simulink library "slib_spectrum_analyser"  (R2020a)
settings: Solver=VariableStepAuto  StartTime=0.0  StopTime=10.0  RelTol=1e-3
libraries: hdlsllib x104, simulink x55, dsphdlxfrm x11, $bdroot x5
(part 1 of 3)
settings Model: Creator=david  LastModifiedBy=kevin

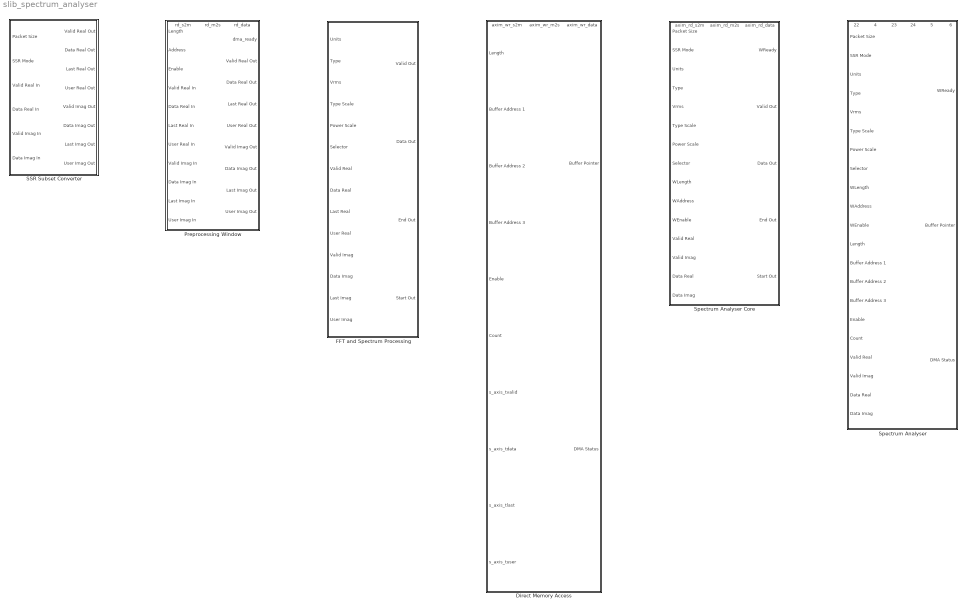
== system slib_spectrum_analyser ==
  Direct Memory Access : Subsystem  TreatAsAtomicUnit=on
      settings: PortSchema="{\"entries\":[{\"content\":{\"sides\":[{\"content\":{\"connectorIds\":[\"In1\",\"In2\",\"In3\",\"In4\",\"In5\",\"In6\",\"In7\",\"In8\",\"In9\",\"In10\"]},\"type\":\"ConnectorPlacement.EquallySpacedRectSide\",\"uuid\":\"feed7d54-868e-4051-a23d-06bc6ab36d5c\"},{\"content\":{\"connectorIds\":[\"Out1\",\"Out2\"],\"side\":\"RIGHT\"},\"type\":\"ConnectorPlacement.EquallySpacedRectSide\",\"uuid\":\"d3d03214-b2fe-4ae7-abfc-e707b28dda07\"},{\"content\":{\"connectorIds\":[\"In11\",\"Out3\",\"Out4\"],\"side\":\"TOP\"},\"type\":\"ConnectorPlacement.EquallySpacedRectSide\",\"uuid\":\"f475a445-5d90-4da5-970d-06e407d01a30\"}]},\"type\":\"ConnectorPlacement.EquallySpacedConnector\",\"uuid\":\"e5023fc6-91ea-4318-839d-5fb8d0ed3484\"}],\"packageUris\":[\"http://schema.mathworks.com/mf0/Connector/19700101\"],\"version\":\"1.0\"}"
  FFT and Spectrum Processing : Subsystem
  Preprocessing Window : Subsystem  TreatAsAtomicUnit=on
      settings: PortSchema="{\"entries\":[{\"content\":{\"sides\":[{\"content\":{\"connectorIds\":[\"In1\",\"In2\",\"In3\",\"In4\",\"In5\",\"In6\",\"In7\",\"In8\",\"In9\",\"In10\",\"In11\"]},\"type\":\"ConnectorPlacement.EquallySpacedRectSide\",\"uuid\":\"9bfde1a4-8e55-439d-ba95-b13ed8c2de82\"},{\"content\":{\"connectorIds\":[\"Out1\",\"Out2\",\"Out3\",\"Out4\",\"Out5\",\"Out6\",\"Out7\",\"Out8\",\"Out9\"],\"side\":\"RIGHT\"},\"type\":\"ConnectorPlacement.EquallySpacedRectSide\",\"uuid\":\"1fa858a7-8a79-448a-a9b9-a47438828a70\"},{\"content\":{\"connectorIds\":[\"In12\",\"Out10\",\"In13\"],\"side\":\"TOP\"},\"type\":\"ConnectorPlacement.EquallySpacedRectSide\",\"uuid\":\"fd991a14-ef2b-4cda-89a6-d580b9713fc0\"}]},\"type\":\"ConnectorPlacement.EquallySpacedConnector\",\"uuid\":\"ee399c2e-0a65-41c3-b55b-7131892126e8\"}],\"packageUris\":[\"http://schema.mathworks.com/mf0/Connector/19700101\"],\"version\":\"1.0\"}"
  SSR Subset Converter : Subsystem  TreatAsAtomicUnit=on
  Spectrum Analyser : Subsystem
      settings: PortSchema="{\"entries\":[{\"content\":{\"sides\":[{\"content\":{\"connectorIds\":[\"In1\",\"In2\",\"In3\",\"In4\",\"In5\",\"In6\",\"In7\",\"In8\",\"In9\",\"In10\",\"In11\",\"In12\",\"In13\",\"In14\",\"In15\",\"In16\",\"In17\",\"In18\",\"In19\",\"In20\",\"In21\"]},\"type\":\"ConnectorPlacement.EquallySpacedRectSide\",\"uuid\":\"d853649d-72ce-4bc9-937e-6765c6958e4b\"},{\"content\":{\"connectorIds\":[\"Out1\",\"Out2\",\"Out3\"],\"side\":\"RIGHT\"},\"type\":\"ConnectorPlacement.EquallySpacedRectSide\",\"uuid\":\"8ee09e61-17e3-46fa-8063-dedf2b48f93c\"},{\"content\":{\"connectorIds\":[\"In22\",\"Out4\",\"In23\",\"In24\",\"Out5\",\"Out6\"],\"side\":\"TOP\"},\"type\":\"ConnectorPlacement.EquallySpacedRectSide\",\"uuid\":\"c9845971-679e-4c10-9868-9337bdd39c3c\"}]},\"type\":\"ConnectorPlacement.EquallySpacedConnector\",\"uuid\":\"5955e85d-b605-4825-a1fe-b5d4f394d259\"}],\"packageUris\":[\"http://schema.mathworks.com/mf0/Connector/19700101\"],\"version\":\"1.0\"}"
  Spectrum Analyser Core : Subsystem
      settings: PortSchema="{\"entries\":[{\"content\":{\"sides\":[{\"content\":{\"connectorIds\":[\"In1\",\"In2\",\"In3\",\"In4\",\"In5\",\"In6\",\"In7\",\"In8\",\"In9\",\"In10\",\"In11\",\"In12\",\"In13\",\"In14\",\"In15\"]},\"type\":\"ConnectorPlacement.EquallySpacedRectSide\",\"uuid\":\"a616570c-2945-48d5-b176-114eb14b1374\"},{\"content\":{\"connectorIds\":[\"Out1\",\"Out2\",\"Out3\",\"Out4\",\"Out5\"],\"side\":\"RIGHT\"},\"type\":\"ConnectorPlacement.EquallySpacedRectSide\",\"uuid\":\"e19b5998-f051-43ca-87c3-ee1f351ddd7e\"},{\"content\":{\"connectorIds\":[\"In16\",\"Out6\",\"In17\"],\"side\":\"TOP\"},\"type\":\"ConnectorPlacement.EquallySpacedRectSide\",\"uuid\":\"3c8ee870-5dc0-4f24-aa51-29f9fa33db38\"}]},\"type\":\"ConnectorPlacement.EquallySpacedConnector\",\"uuid\":\"8f355573-d427-4bf9-9ede-a0a1ced230a6\"}],\"packageUris\":[\"http://schema.mathworks.com/mf0/Connector/19700101\"],\"version\":\"1.0\"}"

== system slib_spectrum_analyser/Direct Memory Access ==
  Length : Inport
  Buffer Address 1 : Inport  Port=2
  Buffer Address 2 : Inport  Port=3
  Buffer Address 3 : Inport  Port=4
  Enable : Inport  Port=5
  Count : Inport  Port=6
  s_axis_tvalid : Inport  Port=7
  s_axis_tdata : Inport  Port=8
  s_axis_tlast : Inport  Port=9
  s_axis_tuser : Inport  Port=10
  axim_wr_s2m : Inport  Port=11
  Direct Memory Access : Subsystem
      settings: PortSchema="{\"entries\":[{\"content\":{\"sides\":[{\"content\":{\"connectorIds\":[\"In1\",\"In2\",\"In3\",\"In4\",\"In5\",\"In6\",\"In7\",\"In8\",\"In9\",\"In10\"]},\"type\":\"ConnectorPlacement.EquallySpacedRectSide\",\"uuid\":\"00536163-74b2-48b0-a433-f45a47e82c13\"},{\"content\":{\"connectorIds\":[\"Out1\",\"Out2\",\"In11\",\"Out3\",\"Out4\",\"Out5\"],\"side\":\"RIGHT\"},\"type\":\"ConnectorPlacement.EquallySpacedRectSide\",\"uuid\":\"bb0450ed-1752-4cb2-9c7c-352c8b1a90c1\"},{\"content\":{\"connectorIds\":[],\"side\":\"TOP\"},\"type\":\"ConnectorPlacement.EquallySpacedRectSide\",\"uuid\":\"451bf01f-2efb-42e7-aace-9484eb9026e5\"}]},\"type\":\"ConnectorPlacement.EquallySpacedConnector\",\"uuid\":\"5c52148d-823b-46a6-a578-8e88341097d4\"}],\"packageUris\":[\"http://schema.mathworks.com/mf0/Connector/19700101\"],\"version\":\"1.0\"}"
  Terminator : Terminator
  Buffer Pointer : Outport
  DMA Status : Outport  Port=2
  axim_wr_m2s : Outport  Port=3
  axim_wr_data : Outport  Port=4
  wires:
  Direct Memory Access/5(debug_signals) -> Terminator/1
  Buffer Address 3/1 -> Direct Memory Access/5(Buffer Address 3)
  Buffer Address 2/1 -> Direct Memory Access/4(Buffer Address 2)
  Length/1 -> Direct Memory Access/1(Length)
  axim_wr_s2m/1 -> Direct Memory Access/11(wr_ready)
  Direct Memory Access/3(Buffer Pointer) -> Buffer Pointer/1
  Direct Memory Access/1(wr_data) -> axim_wr_data/1
  Enable/1 -> Direct Memory Access/6(Enable DMA)
  Buffer Address 1/1 -> Direct Memory Access/3(Buffer Address 1)
  Direct Memory Access/2(wr_m2s) -> axim_wr_m2s/1
  s_axis_tuser/1 -> Direct Memory Access/9(Start In)
  s_axis_tdata/1 -> Direct Memory Access/8(Data In)
  s_axis_tvalid/1 -> Direct Memory Access/7(Valid In)
  s_axis_tlast/1 -> Direct Memory Access/10(End In)
  Count/1 -> Direct Memory Access/2(Count)
  Direct Memory Access/4(DMA Status) -> DMA Status/1

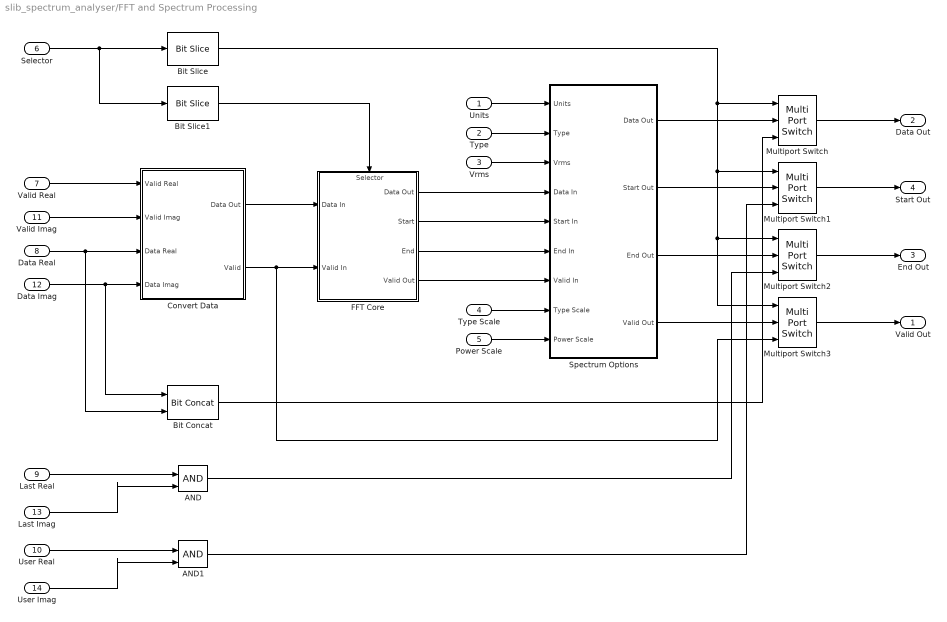
== system slib_spectrum_analyser/FFT and Spectrum Processing ==
  Units : Inport
  Type : Inport  Port=2
  Vrms : Inport  Port=3
  Type Scale : Inport  Port=4
  Power Scale : Inport  Port=5
  Selector : Inport  Port=6
  Valid Real : Inport  Port=7
  Data Real : Inport  Port=8
  Last Real : Inport  Port=9
  User Real : Inport  Port=10
  Valid Imag : Inport  Port=11
  Data Imag : Inport  Port=12
  Last Imag : Inport  Port=13
  User Imag : Inport  Port=14
  AND : Logic  IconShape=distinctive  AllPortsSameDT=off  OutDataTypeStr=boolean
  AND1 : Logic  IconShape=distinctive  AllPortsSameDT=off  OutDataTypeStr=boolean
  Bit Concat : hdlsllib/Logic and Bit Operations/Bit Concat  numInputs=2
  Bit Slice : hdlsllib/Logic and Bit Operations/Bit Slice  lidx=8  ridx=8
      settings: SourceProductBaseCode=SL
  Bit Slice1 : hdlsllib/Logic and Bit Operations/Bit Slice  lidx=7  ridx=0
      settings: SourceProductBaseCode=SL
  Convert Data : Subsystem
  FFT Core : Subsystem  VariantControl=FFT
      settings: PortSchema="{\"entries\":[{\"content\":{\"sides\":[{\"content\":{\"connectorIds\":[\"In1\",\"In2\"]},\"type\":\"ConnectorPlacement.EquallySpacedRectSide\",\"uuid\":\"5a82c6db-67e2-4b0c-874b-00e78ac3fdee\"},{\"content\":{\"connectorIds\":[\"Out1\",\"Out2\",\"Out3\",\"Out4\"],\"side\":\"RIGHT\"},\"type\":\"ConnectorPlacement.EquallySpacedRectSide\",\"uuid\":\"dd11d034-f57b-4257-86c3-a224676007d8\"},{\"content\":{\"connectorIds\":[\"In3\"],\"side\":\"TOP\"},\"type\":\"ConnectorPlacement.EquallySpacedRectSide\",\"uuid\":\"15a5b623-5fad-4b26-a0b8-0856d140e740\"}]},\"type\":\"ConnectorPlacement.EquallySpacedConnector\",\"uuid\":\"f1901d0a-924b-44ce-aa2b-38fba4da21f9\"}],\"packageUris\":[\"http://schema.mathworks.com/mf0/Connector/19700101\"],\"version\":\"1.0\"}"
  Multiport Switch{,1..3} (4 alike) : MultiPortSwitch  DataPortOrder=Zero-based contiguous  Inputs=2  zeroidx=on
  Spectrum Options : Subsystem  VariantControl=Options
  Valid Out : Outport
  Data Out : Outport  Port=2
  End Out : Outport  Port=3
  Start Out : Outport  Port=4
  wires:
  Bit Slice1/1 -> FFT Core/3(Selector)
  Bit Concat/1 -> Multiport Switch/3
  Vrms/1 -> Spectrum Options/3(Vrms)
  User Real/1 -> AND1/1
  Spectrum Options/2(Start Out) -> Multiport Switch1/2
  FFT Core/2(Start) -> Spectrum Options/5(Start In)
  AND/1 -> Multiport Switch2/3
  Spectrum Options/4(Valid Out) -> Multiport Switch3/2
  Last Imag/1 -> AND/2
  Multiport Switch3/1 -> Valid Out/1
  AND1/1 -> Multiport Switch1/3
  Multiport Switch/1 -> Data Out/1
  FFT Core/1(Data Out) -> Spectrum Options/4(Data In)
  Spectrum Options/3(End Out) -> Multiport Switch2/2
  Data Imag/1 -> Convert Data/4(Data Imag), Bit Concat/1
  Valid Real/1 -> Convert Data/1(Valid Real)
  Selector/1 -> Bit Slice/1, Bit Slice1/1
  Multiport Switch2/1 -> End Out/1
  Last Real/1 -> AND/1
  Multiport Switch1/1 -> Start Out/1
  Spectrum Options/1(Data Out) -> Multiport Switch/2
  Type Scale/1 -> Spectrum Options/8(Type Scale)
  Data Real/1 -> Convert Data/3(Data Real), Bit Concat/2
  FFT Core/4(Valid Out) -> Spectrum Options/7(Valid In)
  Power Scale/1 -> Spectrum Options/9(Power Scale)
  Convert Data/1(Data Out) -> FFT Core/1(Data In)
  Type/1 -> Spectrum Options/2(Type)
  User Imag/1 -> AND1/2
  Bit Slice/1 -> Multiport Switch/1, Multiport Switch1/1, Multiport Switch2/1, Multiport Switch3/1
  Units/1 -> Spectrum Options/1(Units)
  Valid Imag/1 -> Convert Data/2(Valid Imag)
  Convert Data/2(Valid) -> FFT Core/2(Valid In), Multiport Switch3/3
  FFT Core/3(End) -> Spectrum Options/6(End In)

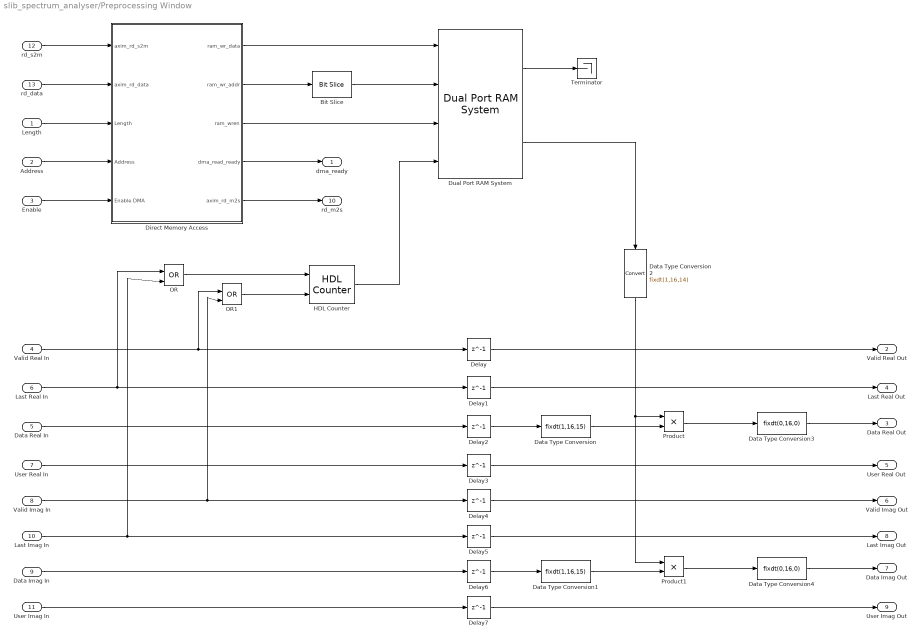
== system slib_spectrum_analyser/Preprocessing Window ==
  Length : Inport
  Address : Inport  Port=2
  Enable : Inport  Port=3
  Valid Real In : Inport  Port=4
  Data Real In : Inport  Port=5
  Last Real In : Inport  Port=6
  User Real In : Inport  Port=7
  Valid Imag In : Inport  Port=8
  Data Imag In : Inport  Port=9
  Last Imag In : Inport  Port=10
  User Imag In : Inport  Port=11
  rd_s2m : Inport  Port=12
  rd_data : Inport  Port=13
  Bit Slice : hdlsllib/Logic and Bit Operations/Bit Slice  lidx=12  ridx=0
      settings: SourceProductBaseCode=SL
  Data Type Conversion : DataTypeConversion  OutDataTypeStr=fixdt(1,16,15)  ConvertRealWorld=Stored Integer (SI)
  Data Type Conversion1 : DataTypeConversion  OutDataTypeStr=fixdt(1,16,15)  ConvertRealWorld=Stored Integer (SI)
  Data Type Conversion2 : DataTypeConversion  OutDataTypeStr=fixdt(1,16,14)  ConvertRealWorld=Stored Integer (SI)
  Data Type Conversion3 : DataTypeConversion  OutDataTypeStr=fixdt(0,16,0)  ConvertRealWorld=Stored Integer (SI)
  Data Type Conversion4 : DataTypeConversion  OutDataTypeStr=fixdt(0,16,0)  ConvertRealWorld=Stored Integer (SI)
  Delay{,1..7} (8 alike) : Delay  DelayLength=1
  Direct Memory Access : Subsystem
  Dual Port RAM System : hdlsllib/HDL RAMs/Dual Port RAM System  RAMType=Dual port  WriteOutputValue=New data  RAMInitialValue=ones(1, 2^13)*2^14  SimulateUsing=Code generation
      settings: SourceProductBaseCode=SL
  HDL Counter : hdlsllib/Sources/HDL Counter  CountType=Count limited  CountInit=0  CountStep=1  CountMax=8191  CountFromType=Initial value  CountFrom=0  CountResetPort=on  CountLoadPort=off  CountEnbPort=on  CountDirPort=off  CountDataType=Unsigned  CountWordLen=13  CountFracLen=0  CountSampTime=1
  OR : Logic  Operator=OR  IconShape=distinctive  AllPortsSameDT=off  OutDataTypeStr=boolean
  OR1 : Logic  Operator=OR  IconShape=distinctive  AllPortsSameDT=off  OutDataTypeStr=boolean
  Product : Product  OutDataTypeStr=fixdt(1,16,15)  RndMeth=Round  SaturateOnIntegerOverflow=on
  Product1 : Product  OutDataTypeStr=fixdt(1,16,15)  RndMeth=Round  SaturateOnIntegerOverflow=on
  Terminator : Terminator
  dma_ready : Outport
  Valid Real Out : Outport  Port=2
  Data Real Out : Outport  Port=3
  Last Real Out : Outport  Port=4
  User Real Out : Outport  Port=5
  Valid Imag Out : Outport  Port=6
  Data Imag Out : Outport  Port=7
  Last Imag Out : Outport  Port=8
  User Imag Out : Outport  Port=9
  rd_m2s : Outport  Port=10
  wires:
  Address/1 -> Direct Memory Access/4(Address)
  Enable/1 -> Direct Memory Access/5(Enable DMA)
  Length/1 -> Direct Memory Access/3(Length)
  Direct Memory Access/1(ram_wr_data) -> Dual Port RAM System/1
  Direct Memory Access/2(ram_wr_addr) -> Bit Slice/1
  Direct Memory Access/3(ram_wren) -> Dual Port RAM System/3
  Direct Memory Access/4(dma_read_ready) -> dma_ready/1
  HDL Counter/1 -> Dual Port RAM System/4
  Valid Real In/1 -> OR1/1, Delay/1
  Last Real In/1 -> OR/1, Delay1/1
  Dual Port RAM System/1 -> Terminator/1
  Direct Memory Access/5(axim_rd_m2s) -> rd_m2s/1
  Dual Port RAM System/2 -> Data Type Conversion2/1
  Data Real In/1 -> Delay2/1
  Product/1 -> Data Type Conversion3/1
  User Real In/1 -> Delay3/1
  OR/1 -> HDL Counter/1
  OR1/1 -> HDL Counter/2
  Last Imag In/1 -> OR/2, Delay5/1
  Valid Imag In/1 -> OR1/2, Delay4/1
  Data Imag In/1 -> Delay6/1
  Product1/1 -> Data Type Conversion4/1
  User Imag In/1 -> Delay7/1
  rd_s2m/1 -> Direct Memory Access/1(axim_rd_s2m)
  rd_data/1 -> Direct Memory Access/2(axim_rd_data)
  Data Type Conversion/1 -> Product/2
  Data Type Conversion1/1 -> Product1/2
  Data Type Conversion2/1 -> Product1/1, Product/1
  Data Type Conversion3/1 -> Data Real Out/1
  Data Type Conversion4/1 -> Data Imag Out/1
  Delay/1 -> Valid Real Out/1
  Delay1/1 -> Last Real Out/1
  Delay2/1 -> Data Type Conversion/1
  Delay3/1 -> User Real Out/1
  Delay4/1 -> Valid Imag Out/1
  Delay5/1 -> Last Imag Out/1
  Delay6/1 -> Data Type Conversion1/1
  Delay7/1 -> User Imag Out/1
  Bit Slice/1 -> Dual Port RAM System/2

== system slib_spectrum_analyser/SSR Subset Converter ==
  Packet Size : Inport
  SSR Mode : Inport  Port=2
  Valid Real In : Inport  Port=3
  Data Real In : Inport  Port=4
  Valid Imag In : Inport  Port=5
  Data Imag In : Inport  Port=6
  Bit Slice : hdlsllib/Logic and Bit Operations/Bit Slice  lidx=3  ridx=0
      settings: SourceProductBaseCode=SL
  SSR Deserializer Imag : Subsystem
  SSR Deserializer Real : Subsystem
  SSR Packet Generator Imag : Subsystem
      settings: PortSchema="{\"entries\":[{\"content\":{\"sides\":[{\"content\":{\"connectorIds\":[\"In1\",\"In2\",\"In3\"]},\"type\":\"ConnectorPlacement.EquallySpacedRectSide\",\"uuid\":\"a59bbe9b-b017-421a-b59e-ccf8f0be8c6c\"},{\"content\":{\"connectorIds\":[\"Out1\",\"Out2\",\"Out3\",\"Out4\"],\"side\":\"RIGHT\"},\"type\":\"ConnectorPlacement.EquallySpacedRectSide\",\"uuid\":\"db28a192-666b-40ba-a3e6-dc552d532719\"},{\"content\":{\"connectorIds\":[\"In4\"],\"side\":\"TOP\"},\"type\":\"ConnectorPlacement.EquallySpacedRectSide\",\"uuid\":\"3e188adb-8196-4c2d-ad94-9c10f40ece47\"}]},\"type\":\"ConnectorPlacement.EquallySpacedConnector\",\"uuid\":\"a5800336-434d-4feb-8784-3c17a141dc8c\"}],\"packageUris\":[\"http://schema.mathworks.com/mf0/Connector/19700101\"],\"version\":\"1.0\"}"
  SSR Packet Generator Real : Subsystem
      settings: PortSchema="{\"entries\":[{\"content\":{\"sides\":[{\"content\":{\"connectorIds\":[\"In1\",\"In2\",\"In3\"]},\"type\":\"ConnectorPlacement.EquallySpacedRectSide\",\"uuid\":\"a59bbe9b-b017-421a-b59e-ccf8f0be8c6c\"},{\"content\":{\"connectorIds\":[\"Out1\",\"Out2\",\"Out3\",\"Out4\"],\"side\":\"RIGHT\"},\"type\":\"ConnectorPlacement.EquallySpacedRectSide\",\"uuid\":\"db28a192-666b-40ba-a3e6-dc552d532719\"},{\"content\":{\"connectorIds\":[\"In4\"],\"side\":\"TOP\"},\"type\":\"ConnectorPlacement.EquallySpacedRectSide\",\"uuid\":\"3e188adb-8196-4c2d-ad94-9c10f40ece47\"}]},\"type\":\"ConnectorPlacement.EquallySpacedConnector\",\"uuid\":\"a5800336-434d-4feb-8784-3c17a141dc8c\"}],\"packageUris\":[\"http://schema.mathworks.com/mf0/Connector/19700101\"],\"version\":\"1.0\"}"
  SSR Serializer Imag : Subsystem
  SSR Serializer Real : Subsystem
  Valid Real Out : Outport
  Data Real Out : Outport  Port=2
  Last Real Out : Outport  Port=3
  User Real Out : Outport  Port=4
  Valid Imag Out : Outport  Port=5
  Data Imag Out : Outport  Port=6
  Last Imag Out : Outport  Port=7
  User Imag Out : Outport  Port=8
  wires:
  SSR Serializer Real/2(Data Out) -> SSR Packet Generator Real/3(Data In)
  SSR Packet Generator Real/4(EoF Out) -> SSR Deserializer Real/4(EoF In)
  Data Real In/1 -> SSR Serializer Real/3(Data In)
  SSR Serializer Real/1(Valid Out) -> SSR Packet Generator Real/2(Valid In)
  SSR Deserializer Real/3(SoF Out) -> User Real Out/1
  Bit Slice/1 -> SSR Serializer Real/1(SSR Control), SSR Serializer Imag/1(SSR Control), SSR Packet Generator Real/1(Frame Drop), SSR Packet Generator Imag/1(Frame Drop)
  SSR Packet Generator Real/1(Valid Out) -> SSR Deserializer Real/1(Valid In)
  Valid Real In/1 -> SSR Serializer Real/2(Valid In)
  SSR Packet Generator Real/3(SoF Out) -> SSR Deserializer Real/3(SoF In)
  SSR Packet Generator Real/2(Data Out) -> SSR Deserializer Real/2(Data In)
  SSR Deserializer Real/2(Data Out) -> Data Real Out/1
  SSR Mode/1 -> Bit Slice/1
  SSR Deserializer Real/1(Valid Out) -> Valid Real Out/1
  SSR Deserializer Real/4(EoL Out) -> Last Real Out/1
  Packet Size/1 -> SSR Packet Generator Real/4(Packet Size), SSR Packet Generator Imag/4(Packet Size)
  Valid Imag In/1 -> SSR Serializer Imag/2(Valid In)
  Data Imag In/1 -> SSR Serializer Imag/3(Data In)
  SSR Serializer Imag/1(Valid Out) -> SSR Packet Generator Imag/2(Valid In)
  SSR Serializer Imag/2(Data Out) -> SSR Packet Generator Imag/3(Data In)
  SSR Deserializer Imag/4(EoL Out) -> Last Imag Out/1
  SSR Deserializer Imag/1(Valid Out) -> Valid Imag Out/1
  SSR Deserializer Imag/2(Data Out) -> Data Imag Out/1
  SSR Deserializer Imag/3(SoF Out) -> User Imag Out/1
  SSR Packet Generator Imag/1(Valid Out) -> SSR Deserializer Imag/1(Valid In)
  SSR Packet Generator Imag/2(Data Out) -> SSR Deserializer Imag/2(Data In)
  SSR Packet Generator Imag/3(SoF Out) -> SSR Deserializer Imag/3(SoF In)
  SSR Packet Generator Imag/4(EoF Out) -> SSR Deserializer Imag/4(EoF In)

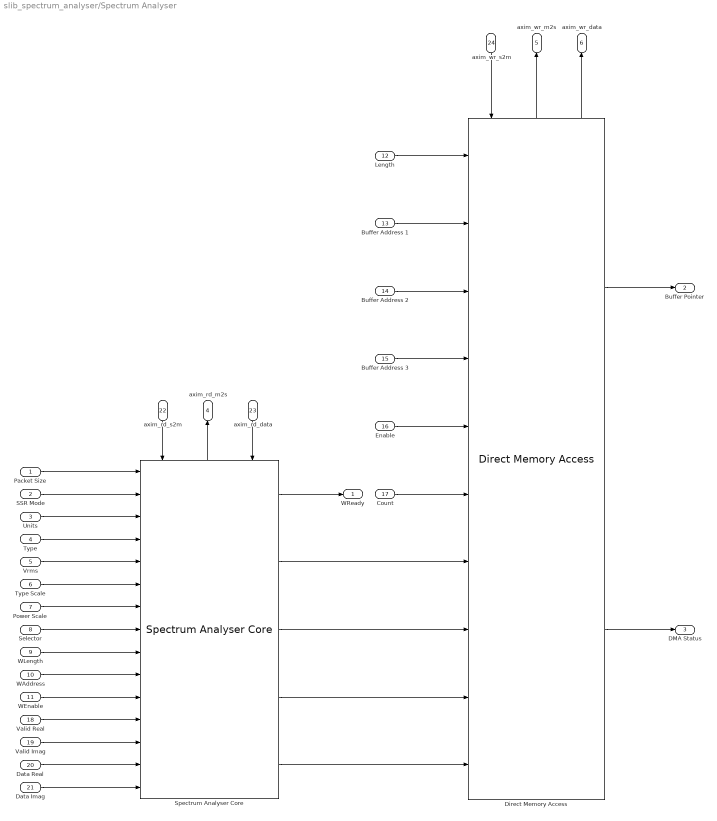
== system slib_spectrum_analyser/Spectrum Analyser ==
  Packet Size : Inport
  SSR Mode : Inport  Port=2
  Units : Inport  Port=3
  Type : Inport  Port=4
  Vrms : Inport  Port=5
  Type Scale : Inport  Port=6
  Power Scale : Inport  Port=7
  Selector : Inport  Port=8
  WLength : Inport  Port=9
  WAddress : Inport  Port=10
  WEnable : Inport  Port=11
  Length : Inport  Port=12
  Buffer Address 1 : Inport  Port=13
  Buffer Address 2 : Inport  Port=14
  Buffer Address 3 : Inport  Port=15
  Enable : Inport  Port=16
  Count : Inport  Port=17
  Valid Real : Inport  Port=18
  Valid Imag : Inport  Port=19
  Data Real : Inport  Port=20
  Data Imag : Inport  Port=21
  axim_rd_s2m : Inport  Port=22
  axim_rd_data : Inport  Port=23
  axim_wr_s2m : Inport  Port=24
  Direct Memory Access : $bdroot/Direct Memory Access  SystemSampleTime=-1  Latency=0  AutoFrameSizeCalculation=off
      settings: PortSchema="{\"entries\":[{\"content\":{\"sides\":[{\"content\":{\"connectorIds\":[\"In1\",\"In2\",\"In3\",\"In4\",\"In5\",\"In6\",\"In7\",\"In8\",\"In9\",\"In10\"]},\"type\":\"ConnectorPlacement.EquallySpacedRectSide\",\"uuid\":\"feed7d54-868e-4051-a23d-06bc6ab36d5c\"},{\"content\":{\"connectorIds\":[\"Out1\",\"Out2\"],\"side\":\"RIGHT\"},\"type\":\"ConnectorPlacement.EquallySpacedRectSide\",\"uuid\":\"d3d03214-b2fe-4ae7-abfc-e707b28dda07\"},{\"content\":{\"connectorIds\":[\"In11\",\"Out3\",\"Out4\"],\"side\":\"TOP\"},\"type\":\"ConnectorPlacement.EquallySpacedRectSide\",\"uuid\":\"f475a445-5d90-4da5-970d-06e407d01a30\"}]},\"type\":\"ConnectorPlacement.EquallySpacedConnector\",\"uuid\":\"e5023fc6-91ea-4318-839d-5fb8d0ed3484\"}],\"packageUris\":[\"http://schema.mathworks.com/mf0/Connector/19700101\"],\"version\":\"1.0\"}"
  Spectrum Analyser Core : $bdroot/Spectrum Analyser Core  SystemSampleTime=-1  Latency=0  AutoFrameSizeCalculation=off
      settings: PortSchema="{\"entries\":[{\"content\":{\"sides\":[{\"content\":{\"connectorIds\":[\"In1\",\"In2\",\"In3\",\"In4\",\"In5\",\"In6\",\"In7\",\"In8\",\"In9\",\"In10\",\"In11\",\"In12\",\"In13\",\"In14\",\"In15\"]},\"type\":\"ConnectorPlacement.EquallySpacedRectSide\",\"uuid\":\"a616570c-2945-48d5-b176-114eb14b1374\"},{\"content\":{\"connectorIds\":[\"Out1\",\"Out2\",\"Out3\",\"Out4\",\"Out5\"],\"side\":\"RIGHT\"},\"type\":\"ConnectorPlacement.EquallySpacedRectSide\",\"uuid\":\"e19b5998-f051-43ca-87c3-ee1f351ddd7e\"},{\"content\":{\"connectorIds\":[\"In16\",\"Out6\",\"In17\"],\"side\":\"TOP\"},\"type\":\"ConnectorPlacement.EquallySpacedRectSide\",\"uuid\":\"3c8ee870-5dc0-4f24-aa51-29f9fa33db38\"}]},\"type\":\"ConnectorPlacement.EquallySpacedConnector\",\"uuid\":\"8f355573-d427-4bf9-9ede-a0a1ced230a6\"}],\"packageUris\":[\"http://schema.mathworks.com/mf0/Connector/19700101\"],\"version\":\"1.0\"}"
  WReady : Outport
  Buffer Pointer : Outport  Port=2
  DMA Status : Outport  Port=3
  axim_rd_m2s : Outport  Port=4
  axim_wr_m2s : Outport  Port=5
  axim_wr_data : Outport  Port=6
  wires:
  Direct Memory Access/3 -> axim_wr_m2s/1
  Spectrum Analyser Core/5 -> Direct Memory Access/10
  Spectrum Analyser Core/4 -> Direct Memory Access/9
  axim_rd_data/1 -> Spectrum Analyser Core/17
  Spectrum Analyser Core/3 -> Direct Memory Access/8
  Enable/1 -> Direct Memory Access/5
  axim_rd_s2m/1 -> Spectrum Analyser Core/16
  Spectrum Analyser Core/2 -> Direct Memory Access/7
  WEnable/1 -> Spectrum Analyser Core/11
  Data Imag/1 -> Spectrum Analyser Core/15
  Units/1 -> Spectrum Analyser Core/3
  WAddress/1 -> Spectrum Analyser Core/10
  Spectrum Analyser Core/1 -> WReady/1
  Power Scale/1 -> Spectrum Analyser Core/7
  Buffer Address 1/1 -> Direct Memory Access/2
  Type Scale/1 -> Spectrum Analyser Core/6
  Valid Real/1 -> Spectrum Analyser Core/12
  WLength/1 -> Spectrum Analyser Core/9
  Selector/1 -> Spectrum Analyser Core/8
  Type/1 -> Spectrum Analyser Core/4
  axim_wr_s2m/1 -> Direct Memory Access/11
  Direct Memory Access/4 -> axim_wr_data/1
  Packet Size/1 -> Spectrum Analyser Core/1
  Data Real/1 -> Spectrum Analyser Core/14
  Buffer Address 3/1 -> Direct Memory Access/4
  Direct Memory Access/2 -> DMA Status/1
  Direct Memory Access/1 -> Buffer Pointer/1
  Count/1 -> Direct Memory Access/6
  Spectrum Analyser Core/6 -> axim_rd_m2s/1
  Buffer Address 2/1 -> Direct Memory Access/3
  Length/1 -> Direct Memory Access/1
  SSR Mode/1 -> Spectrum Analyser Core/2
  Vrms/1 -> Spectrum Analyser Core/5
  Valid Imag/1 -> Spectrum Analyser Core/13

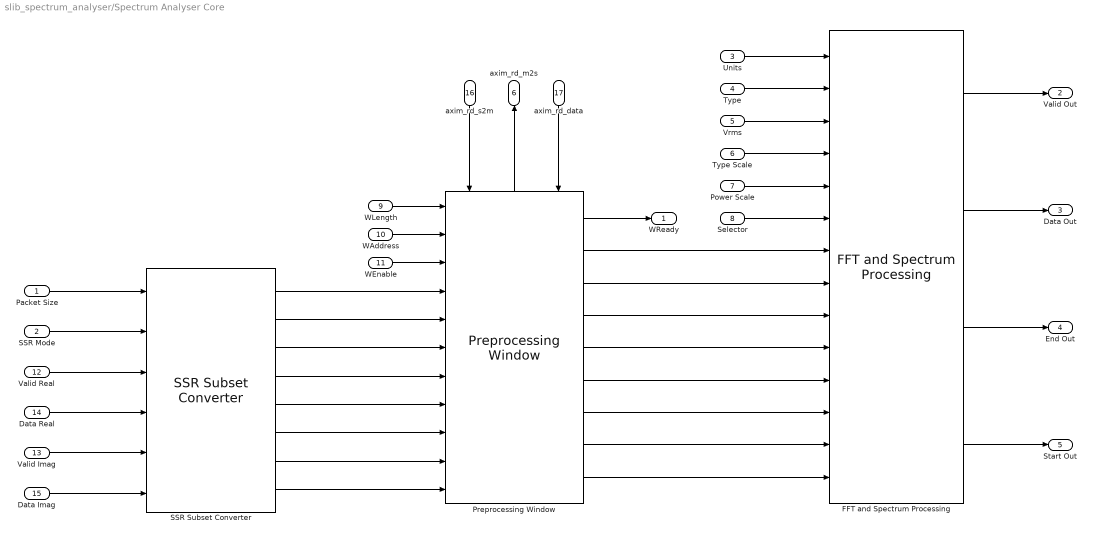
== system slib_spectrum_analyser/Spectrum Analyser Core ==
  Packet Size : Inport
  SSR Mode : Inport  Port=2
  Units : Inport  Port=3
  Type : Inport  Port=4
  Vrms : Inport  Port=5
  Type Scale : Inport  Port=6
  Power Scale : Inport  Port=7
  Selector : Inport  Port=8
  WLength : Inport  Port=9
  WAddress : Inport  Port=10
  WEnable : Inport  Port=11
  Valid Real : Inport  Port=12
  Valid Imag : Inport  Port=13
  Data Real : Inport  Port=14
  Data Imag : Inport  Port=15
  axim_rd_s2m : Inport  Port=16
  axim_rd_data : Inport  Port=17
  FFT and Spectrum Processing : $bdroot/FFT and Spectrum Processing  SystemSampleTime=-1  Latency=0  AutoFrameSizeCalculation=off
  Preprocessing Window : $bdroot/Preprocessing Window  SystemSampleTime=-1  Latency=0  AutoFrameSizeCalculation=off
      settings: PortSchema="{\"entries\":[{\"content\":{\"sides\":[{\"content\":{\"connectorIds\":[\"In1\",\"In2\",\"In3\",\"In4\",\"In5\",\"In6\",\"In7\",\"In8\",\"In9\",\"In10\",\"In11\"]},\"type\":\"ConnectorPlacement.EquallySpacedRectSide\",\"uuid\":\"9bfde1a4-8e55-439d-ba95-b13ed8c2de82\"},{\"content\":{\"connectorIds\":[\"Out1\",\"Out2\",\"Out3\",\"Out4\",\"Out5\",\"Out6\",\"Out7\",\"Out8\",\"Out9\"],\"side\":\"RIGHT\"},\"type\":\"ConnectorPlacement.EquallySpacedRectSide\",\"uuid\":\"1fa858a7-8a79-448a-a9b9-a47438828a70\"},{\"content\":{\"connectorIds\":[\"In12\",\"Out10\",\"In13\"],\"side\":\"TOP\"},\"type\":\"ConnectorPlacement.EquallySpacedRectSide\",\"uuid\":\"fd991a14-ef2b-4cda-89a6-d580b9713fc0\"}]},\"type\":\"ConnectorPlacement.EquallySpacedConnector\",\"uuid\":\"ee399c2e-0a65-41c3-b55b-7131892126e8\"}],\"packageUris\":[\"http://schema.mathworks.com/mf0/Connector/19700101\"],\"version\":\"1.0\"}"
  SSR Subset Converter : $bdroot/SSR Subset Converter  SystemSampleTime=-1  Latency=0  AutoFrameSizeCalculation=off
  WReady : Outport
  Valid Out : Outport  Port=2
  Data Out : Outport  Port=3
  End Out : Outport  Port=4
  Start Out : Outport  Port=5
  axim_rd_m2s : Outport  Port=6
  wires:
  Valid Imag/1 -> SSR Subset Converter/5
  Preprocessing Window/5 -> FFT and Spectrum Processing/10
  Preprocessing Window/1 -> WReady/1
  SSR Subset Converter/7 -> Preprocessing Window/10
  WEnable/1 -> Preprocessing Window/3
  Valid Real/1 -> SSR Subset Converter/3
  SSR Subset Converter/6 -> Preprocessing Window/9
  FFT and Spectrum Processing/2 -> Data Out/1
  axim_rd_data/1 -> Preprocessing Window/13
  Units/1 -> FFT and Spectrum Processing/1
  Preprocessing Window/8 -> FFT and Spectrum Processing/13
  FFT and Spectrum Processing/1 -> Valid Out/1
  Preprocessing Window/6 -> FFT and Spectrum Processing/11
  SSR Subset Converter/3 -> Preprocessing Window/6
  axim_rd_s2m/1 -> Preprocessing Window/12
  SSR Subset Converter/8 -> Preprocessing Window/11
  WLength/1 -> Preprocessing Window/1
  FFT and Spectrum Processing/3 -> End Out/1
  Data Real/1 -> SSR Subset Converter/4
  Preprocessing Window/7 -> FFT and Spectrum Processing/12
  SSR Mode/1 -> SSR Subset Converter/2
  Data Imag/1 -> SSR Subset Converter/6
  SSR Subset Converter/4 -> Preprocessing Window/7
  Power Scale/1 -> FFT and Spectrum Processing/5
  Preprocessing Window/4 -> FFT and Spectrum Processing/9
  SSR Subset Converter/5 -> Preprocessing Window/8
  Type/1 -> FFT and Spectrum Processing/2
  Vrms/1 -> FFT and Spectrum Processing/3
  Preprocessing Window/2 -> FFT and Spectrum Processing/7
  Selector/1 -> FFT and Spectrum Processing/6
  FFT and Spectrum Processing/4 -> Start Out/1
  Type Scale/1 -> FFT and Spectrum Processing/4
  WAddress/1 -> Preprocessing Window/2
  SSR Subset Converter/2 -> Preprocessing Window/5
  Preprocessing Window/9 -> FFT and Spectrum Processing/14
  Preprocessing Window/10 -> axim_rd_m2s/1
  SSR Subset Converter/1 -> Preprocessing Window/4
  Preprocessing Window/3 -> FFT and Spectrum Processing/8
  Packet Size/1 -> SSR Subset Converter/1

== system slib_spectrum_analyser/Direct Memory Access/Direct Memory Access ==
  Length : Inport
  Count : Inport  Port=2
  Buffer Address 1 : Inport  Port=3
  Buffer Address 2 : Inport  Port=4
  Buffer Address 3 : Inport  Port=5
  Enable DMA : Inport  Port=6
  Valid In : Inport  Port=7
  Data In : Inport  Port=8
  Start In : Inport  Port=9
  End In : Inport  Port=10
  wr_ready : Inport  Port=11
  DDR Communication : Subsystem
      settings: PortSchema="{\"entries\":[{\"content\":{\"sides\":[{\"content\":{\"connectorIds\":[\"In1\",\"In2\",\"In3\",\"In4\",\"In5\",\"In6\",\"In7\",\"In8\",\"In9\",\"In10\"]},\"type\":\"ConnectorPlacement.EquallySpacedRectSide\",\"uuid\":\"1b0605ed-f994-4b4f-952c-c7a4534a55db\"},{\"content\":{\"connectorIds\":[\"Out1\",\"Out2\",\"Out3\",\"Out4\",\"Out5\",\"In11\"],\"side\":\"RIGHT\"},\"type\":\"ConnectorPlacement.EquallySpacedRectSide\",\"uuid\":\"e00ce3f0-150b-4c4f-a18d-f280380b0728\"},{\"content\":{\"connectorIds\":[],\"side\":\"TOP\"},\"type\":\"ConnectorPlacement.EquallySpacedRectSide\",\"uuid\":\"b0ef8b1e-3f6b-405f-8824-c1fb25b076ef\"}]},\"type\":\"ConnectorPlacement.EquallySpacedConnector\",\"uuid\":\"53c75551-9c59-440c-835f-2065b8683bc1\"}],\"packageUris\":[\"http://schema.mathworks.com/mf0/Connector/19700101\"],\"version\":\"1.0\"}"
  wr_data : Outport
  wr_m2s : Outport  Port=2
  Buffer Pointer : Outport  Port=3
  DMA Status : Outport  Port=4
  debug_signals : Outport  Port=5
  wires:
  wr_ready/1 -> DDR Communication/11(wr_ready)
  DDR Communication/2(wr_data) -> wr_data/1
  DDR Communication/3(wr_m2s) -> wr_m2s/1
  Start In/1 -> DDR Communication/9(Start In)
  End In/1 -> DDR Communication/10(End In)
  Data In/1 -> DDR Communication/8(Data Out)
  DDR Communication/1(Buffer Pointer) -> Buffer Pointer/1
  Valid In/1 -> DDR Communication/7(Valid Out)
  Buffer Address 1/1 -> DDR Communication/3(Buffer Address 1)
  Buffer Address 2/1 -> DDR Communication/4(Buffer Address 2)
  Buffer Address 3/1 -> DDR Communication/5(Buffer Address 3)
  Enable DMA/1 -> DDR Communication/6(Enable)
  DDR Communication/4(DMA Status) -> DMA Status/1
  Length/1 -> DDR Communication/1(Length)
  DDR Communication/5(debug_signals) -> debug_signals/1
  Count/1 -> DDR Communication/2(Count)

== system slib_spectrum_analyser/FFT and Spectrum Processing/Convert Data ==
  Valid Real : Inport
  Valid Imag : Inport  Port=2
  Data Real : Inport  Port=3
  Data Imag : Inport  Port=4
  AND : Logic  IconShape=distinctive  AllPortsSameDT=off  OutDataTypeStr=boolean
  Data Type Conversion : DataTypeConversion  OutDataTypeStr=fixdt(1,16,15)  ConvertRealWorld=Stored Integer (SI)
  Data Type Conversion1 : DataTypeConversion  OutDataTypeStr=fixdt(1,16,15)  ConvertRealWorld=Stored Integer (SI)
  Real-Imag to Complex : RealImagToComplex
  Data Out : Outport
  Valid : Outport  Port=2
  wires:
  Valid Imag/1 -> AND/2
  Data Type Conversion1/1 -> Real-Imag to Complex/2
  Data Real/1 -> Data Type Conversion/1
  Data Type Conversion/1 -> Real-Imag to Complex/1
  Data Imag/1 -> Data Type Conversion1/1
  Valid Real/1 -> AND/1
  AND/1 -> Valid/1
  Real-Imag to Complex/1 -> Data Out/1

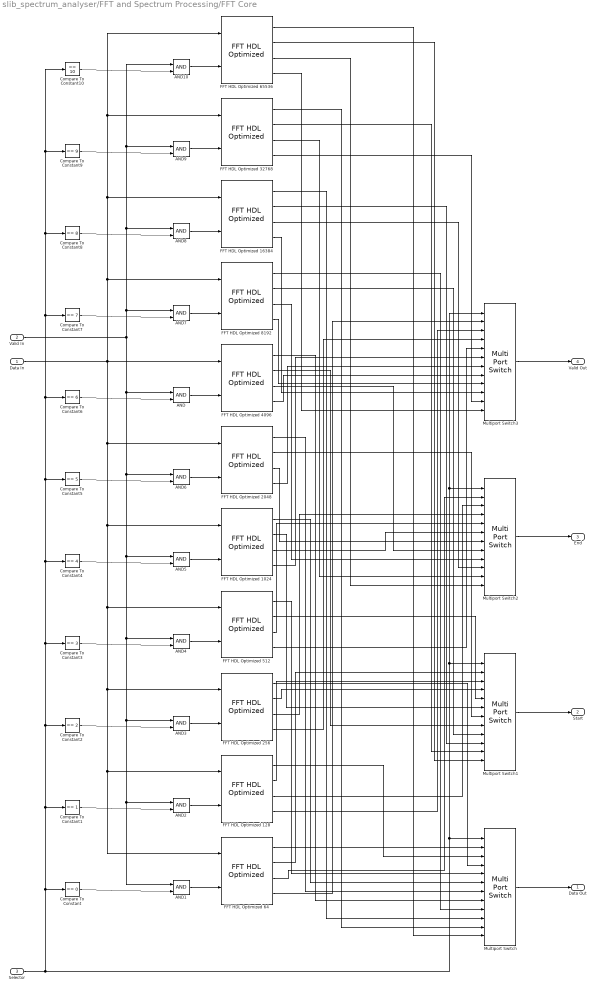
== system slib_spectrum_analyser/FFT and Spectrum Processing/FFT Core ==
  Data In : Inport
  Valid In : Inport  Port=2
  Selector : Inport  Port=3
  AND{,1..10} (11 alike) : Logic  IconShape=distinctive  AllPortsSameDT=off  OutDataTypeStr=boolean
  Compare To Constant : simulink/Logic and Bit Operations/Compare To Constant  relop===  const=0  OutDataTypeStr=boolean
  Compare To Constant1 : simulink/Logic and Bit Operations/Compare To Constant  relop===  const=1  OutDataTypeStr=boolean
  Compare To Constant10 : simulink/Logic and Bit Operations/Compare To Constant  relop===  const=10  OutDataTypeStr=boolean
  Compare To Constant2 : simulink/Logic and Bit Operations/Compare To Constant  relop===  const=2  OutDataTypeStr=boolean
  Compare To Constant3 : simulink/Logic and Bit Operations/Compare To Constant  relop===  const=3  OutDataTypeStr=boolean
  Compare To Constant4 : simulink/Logic and Bit Operations/Compare To Constant  relop===  const=4  OutDataTypeStr=boolean
  Compare To Constant5 : simulink/Logic and Bit Operations/Compare To Constant  relop===  const=5  OutDataTypeStr=boolean
  Compare To Constant6 : simulink/Logic and Bit Operations/Compare To Constant  relop===  const=6  OutDataTypeStr=boolean
  Compare To Constant7 : simulink/Logic and Bit Operations/Compare To Constant  relop===  const=7  OutDataTypeStr=boolean
  Compare To Constant8 : simulink/Logic and Bit Operations/Compare To Constant  relop===  const=8  OutDataTypeStr=boolean
  Compare To Constant9 : simulink/Logic and Bit Operations/Compare To Constant  relop===  const=9  OutDataTypeStr=boolean
  FFT HDL Optimized 1024 : dsphdlxfrm/FFT HDL Optimized  FFTLength=1024  Architecture=Streaming Radix 2^2  ComplexMultiplication=Use 4 multipliers and 2 adders  BitReversedOutput=off  BitReversedInput=off  Normalize=off  SimulateUsing=Code generation  RoundingMethod=Round  ResetInputPort=off  StartOutputPort=on  EndOutputPort=on
      settings: SourceProductBaseCode=DS
  FFT HDL Optimized 128 : dsphdlxfrm/FFT HDL Optimized  FFTLength=128  Architecture=Streaming Radix 2^2  ComplexMultiplication=Use 4 multipliers and 2 adders  BitReversedOutput=off  BitReversedInput=off  Normalize=off  SimulateUsing=Code generation  RoundingMethod=Round  ResetInputPort=off  StartOutputPort=on  EndOutputPort=on
      settings: SourceProductBaseCode=DS
  FFT HDL Optimized 16384 : dsphdlxfrm/FFT HDL Optimized  FFTLength=16384  Architecture=Streaming Radix 2^2  ComplexMultiplication=Use 4 multipliers and 2 adders  BitReversedOutput=off  BitReversedInput=off  Normalize=off  SimulateUsing=Code generation  RoundingMethod=Round  ResetInputPort=off  StartOutputPort=on  EndOutputPort=on
      settings: SourceProductBaseCode=DS
  FFT HDL Optimized 2048 : dsphdlxfrm/FFT HDL Optimized  FFTLength=2048  Architecture=Streaming Radix 2^2  ComplexMultiplication=Use 4 multipliers and 2 adders  BitReversedOutput=off  BitReversedInput=off  Normalize=off  SimulateUsing=Code generation  RoundingMethod=Round  ResetInputPort=off  StartOutputPort=on  EndOutputPort=on
      settings: SourceProductBaseCode=DS
  FFT HDL Optimized 256 : dsphdlxfrm/FFT HDL Optimized  FFTLength=256  Architecture=Streaming Radix 2^2  ComplexMultiplication=Use 4 multipliers and 2 adders  BitReversedOutput=off  BitReversedInput=off  Normalize=off  SimulateUsing=Code generation  RoundingMethod=Round  ResetInputPort=off  StartOutputPort=on  EndOutputPort=on
      settings: SourceProductBaseCode=DS
  FFT HDL Optimized 32768 : dsphdlxfrm/FFT HDL Optimized  FFTLength=32768  Architecture=Streaming Radix 2^2  ComplexMultiplication=Use 4 multipliers and 2 adders  BitReversedOutput=off  BitReversedInput=off  Normalize=off  SimulateUsing=Code generation  RoundingMethod=Round  ResetInputPort=off  StartOutputPort=on  EndOutputPort=on
      settings: SourceProductBaseCode=DS
  FFT HDL Optimized 4096 : dsphdlxfrm/FFT HDL Optimized  FFTLength=4096  Architecture=Streaming Radix 2^2  ComplexMultiplication=Use 4 multipliers and 2 adders  BitReversedOutput=off  BitReversedInput=off  Normalize=off  SimulateUsing=Code generation  RoundingMethod=Round  ResetInputPort=off  StartOutputPort=on  EndOutputPort=on
      settings: SourceProductBaseCode=DS
  FFT HDL Optimized 512 : dsphdlxfrm/FFT HDL Optimized  FFTLength=512  Architecture=Streaming Radix 2^2  ComplexMultiplication=Use 4 multipliers and 2 adders  BitReversedOutput=off  BitReversedInput=off  Normalize=off  SimulateUsing=Code generation  RoundingMethod=Round  ResetInputPort=off  StartOutputPort=on  EndOutputPort=on
      settings: SourceProductBaseCode=DS
  FFT HDL Optimized 64 : dsphdlxfrm/FFT HDL Optimized  FFTLength=64  Architecture=Streaming Radix 2^2  ComplexMultiplication=Use 4 multipliers and 2 adders  BitReversedOutput=off  BitReversedInput=off  Normalize=off  SimulateUsing=Code generation  RoundingMethod=Round  ResetInputPort=off  StartOutputPort=on  EndOutputPort=on
      settings: SourceProductBaseCode=DS
  FFT HDL Optimized 65536 : dsphdlxfrm/FFT HDL Optimized  FFTLength=65536  Architecture=Streaming Radix 2^2  ComplexMultiplication=Use 4 multipliers and 2 adders  BitReversedOutput=off  BitReversedInput=off  Normalize=off  SimulateUsing=Code generation  RoundingMethod=Round  ResetInputPort=off  StartOutputPort=on  EndOutputPort=on
      settings: SourceProductBaseCode=DS
  FFT HDL Optimized 8192 : dsphdlxfrm/FFT HDL Optimized  FFTLength=8192  Architecture=Streaming Radix 2^2  ComplexMultiplication=Use 4 multipliers and 2 adders  BitReversedOutput=off  BitReversedInput=off  Normalize=off  SimulateUsing=Code generation  RoundingMethod=Round  ResetInputPort=off  StartOutputPort=on  EndOutputPort=on
      settings: SourceProductBaseCode=DS
  Multiport Switch{,1..3} (4 alike) : MultiPortSwitch  DataPortOrder=Zero-based contiguous  Inputs=11  zeroidx=on
  Data Out : Outport
  Start : Outport  Port=2
  End : Outport  Port=3
  Valid Out : Outport  Port=4
  wires:
  Multiport Switch/1 -> Data Out/1
  Multiport Switch1/1 -> Start/1
  Multiport Switch2/1 -> End/1
  Multiport Switch3/1 -> Valid Out/1
  FFT HDL Optimized 64/4 -> Multiport Switch3/2
  FFT HDL Optimized 128/4 -> Multiport Switch3/3
  FFT HDL Optimized 256/4 -> Multiport Switch3/4
  FFT HDL Optimized 512/4 -> Multiport Switch3/5
  FFT HDL Optimized 1024/4 -> Multiport Switch3/6
  FFT HDL Optimized 2048/4 -> Multiport Switch3/7
  FFT HDL Optimized 8192/4 -> Multiport Switch3/9
  FFT HDL Optimized 4096/4 -> Multiport Switch3/8
  FFT HDL Optimized 64/3 -> Multiport Switch2/2
  FFT HDL Optimized 128/3 -> Multiport Switch2/3
  FFT HDL Optimized 8192/3 -> Multiport Switch2/9
  FFT HDL Optimized 4096/3 -> Multiport Switch2/8
  FFT HDL Optimized 2048/3 -> Multiport Switch2/7
  FFT HDL Optimized 256/3 -> Multiport Switch2/4
  FFT HDL Optimized 512/3 -> Multiport Switch2/5
  FFT HDL Optimized 1024/3 -> Multiport Switch2/6
  FFT HDL Optimized 8192/2 -> Multiport Switch1/9
  FFT HDL Optimized 4096/2 -> Multiport Switch1/8
  FFT HDL Optimized 2048/2 -> Multiport Switch1/7
  FFT HDL Optimized 1024/2 -> Multiport Switch1/6
  FFT HDL Optimized 512/2 -> Multiport Switch1/5
  FFT HDL Optimized 128/2 -> Multiport Switch1/3
  FFT HDL Optimized 64/2 -> Multiport Switch1/2
  FFT HDL Optimized 256/2 -> Multiport Switch1/4
  FFT HDL Optimized 8192/1 -> Multiport Switch/9
  FFT HDL Optimized 4096/1 -> Multiport Switch/8
  FFT HDL Optimized 2048/1 -> Multiport Switch/7
  FFT HDL Optimized 1024/1 -> Multiport Switch/6
  FFT HDL Optimized 512/1 -> Multiport Switch/5
  FFT HDL Optimized 256/1 -> Multiport Switch/4
  FFT HDL Optimized 128/1 -> Multiport Switch/3
  FFT HDL Optimized 64/1 -> Multiport Switch/2
  Compare To Constant6/1 -> AND/2
  Compare To Constant5/1 -> AND6/2
  Compare To Constant4/1 -> AND5/2
  Compare To Constant3/1 -> AND4/2
  Compare To Constant2/1 -> AND3/2
  Compare To Constant1/1 -> AND2/2
  Data In/1 -> FFT HDL Optimized 65536/1, FFT HDL Optimized 32768/1, FFT HDL Optimized 16384/1, FFT HDL Optimized 8192/1, FFT HDL Optimized 4096/1, FFT HDL Optimized 2048/1, FFT HDL Optimized 1024/1, FFT HDL Optimized 512/1, FFT HDL Optimized 256/1, FFT HDL Optimized 128/1, FFT HDL Optimized 64/1
  Compare To Constant7/1 -> AND7/2
  AND7/1 -> FFT HDL Optimized 8192/2
  AND6/1 -> FFT HDL Optimized 2048/2
  AND5/1 -> FFT HDL Optimized 1024/2
  AND4/1 -> FFT HDL Optimized 512/2
  AND2/1 -> FFT HDL Optimized 128/2
  AND3/1 -> FFT HDL Optimized 256/2
  Valid In/1 -> AND7/1, AND10/1, AND9/1, AND8/1, AND1/1, AND2/1, AND3/1, AND4/1, AND5/1, AND6/1, AND/1
  Selector/1 -> Compare To Constant/1, Compare To Constant1/1, Compare To Constant2/1, Compare To Constant3/1, Compare To Constant4/1, Compare To Constant5/1, Compare To Constant6/1, Compare To Constant10/1, Compare To Constant9/1, Compare To Constant8/1, Compare To Constant7/1, Multiport Switch3/1, Multiport Switch2/1, Multiport Switch1/1, Multiport Switch/1
  Compare To Constant/1 -> AND1/2
  AND1/1 -> FFT HDL Optimized 64/2
  AND/1 -> FFT HDL Optimized 4096/2
  FFT HDL Optimized 16384/4 -> Multiport Switch3/10
  FFT HDL Optimized 16384/3 -> Multiport Switch2/10
  FFT HDL Optimized 16384/2 -> Multiport Switch1/10
  FFT HDL Optimized 16384/1 -> Multiport Switch/10
  AND8/1 -> FFT HDL Optimized 16384/2
  Compare To Constant8/1 -> AND8/2
  AND9/1 -> FFT HDL Optimized 32768/2
  Compare To Constant9/1 -> AND9/2
  AND10/1 -> FFT HDL Optimized 65536/2
  Compare To Constant10/1 -> AND10/2
  FFT HDL Optimized 32768/4 -> Multiport Switch3/11
  FFT HDL Optimized 32768/3 -> Multiport Switch2/11
  FFT HDL Optimized 32768/2 -> Multiport Switch1/11
  FFT HDL Optimized 32768/1 -> Multiport Switch/11
  FFT HDL Optimized 65536/4 -> Multiport Switch3/12
  FFT HDL Optimized 65536/3 -> Multiport Switch2/12
  FFT HDL Optimized 65536/2 -> Multiport Switch1/12
  FFT HDL Optimized 65536/1 -> Multiport Switch/12

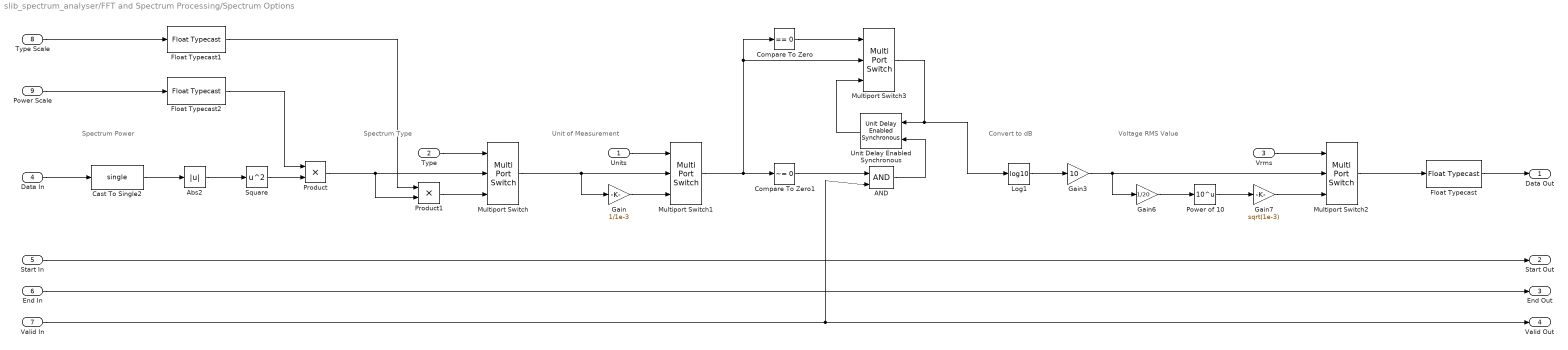
== system slib_spectrum_analyser/FFT and Spectrum Processing/Spectrum Options ==
  note: Voltage RMS Value
  note: Convert to dB
  note: Unit of Measurement
  note: Spectrum Type
  note: Spectrum Power
  Units : Inport
  Type : Inport  Port=2
  Vrms : Inport  Port=3
  Data In : Inport  Port=4
  Start In : Inport  Port=5
  End In : Inport  Port=6
  Valid In : Inport  Port=7
  Type Scale : Inport  Port=8
  Power Scale : Inport  Port=9
  AND : Logic  IconShape=distinctive  AllPortsSameDT=off  OutDataTypeStr=boolean
  Abs2 : Abs
  Cast To Single2 : DataTypeConversion  OutDataTypeStr=single
  Compare To Zero : simulink/Logic and Bit Operations/Compare To Zero  relop===  OutDataTypeStr=boolean
  Compare To Zero1 : simulink/Logic and Bit Operations/Compare To Zero  relop=~=  OutDataTypeStr=boolean
  Float Typecast : FloatTypecast
  Float Typecast1 : FloatTypecast
  Float Typecast2 : FloatTypecast
  Gain : Gain  Gain=1/1e-3
  Gain3 : Gain  Gain=10  ParamDataTypeStr=single  OutDataTypeStr=single
  Gain6 : Gain  Gain=1/20
  Gain7 : Gain  Gain=sqrt(1e-3)
  Log1 : Math  Operator=log10  SignedPower=on  SaturateOnIntegerOverflow=on
  Multiport Switch{,1..3} (4 alike) : MultiPortSwitch  DataPortOrder=Zero-based contiguous  Inputs=2  zeroidx=on
  Power of 10 : Math  Operator=10^u  SaturateOnIntegerOverflow=on
  Product : Product
  Product1 : Product
  Square : Math  Operator=square  SaturateOnIntegerOverflow=on
  Unit Delay Enabled Synchronous : hdlsllib/Discrete/Unit Delay Enabled Synchronous  InitialCondition=0.0  SampleTime=-1
      settings: SourceProductBaseCode=SL
  Data Out : Outport
  Start Out : Outport  Port=2
  End Out : Outport  Port=3
  Valid Out : Outport  Port=4
  wires:
  Float Typecast2/1 -> Product/1
  Float Typecast1/1 -> Product1/1
  Power Scale/1 -> Float Typecast2/1
  Type Scale/1 -> Float Typecast1/1
  Square/1 -> Product/2
  Abs2/1 -> Square/1
  Product/1 -> Multiport Switch/2, Product1/2
  Data In/1 -> Cast To Single2/1
  Cast To Single2/1 -> Abs2/1
  Start In/1 -> Start Out/1
  Log1/1 -> Gain3/1
  Multiport Switch/1 -> Multiport Switch1/2, Gain/1
  Gain6/1 -> Power of 10/1
  Power of 10/1 -> Gain7/1
  Gain3/1 -> Multiport Switch2/2, Gain6/1
  Multiport Switch2/1 -> Float Typecast/1
  Gain7/1 -> Multiport Switch2/3
  Gain/1 -> Multiport Switch1/3
  Product1/1 -> Multiport Switch/3
  Type/1 -> Multiport Switch/1
  Units/1 -> Multiport Switch1/1
  Vrms/1 -> Multiport Switch2/1
  Float Typecast/1 -> Data Out/1
  Valid In/1 -> AND/2, Valid Out/1
  Multiport Switch3/1 -> Log1/1, Unit Delay Enabled Synchronous/1
  Unit Delay Enabled Synchronous/1 -> Multiport Switch3/3
  Compare To Zero/1 -> Multiport Switch3/1
  Compare To Zero1/1 -> AND/1
  AND/1 -> Unit Delay Enabled Synchronous/2
  End In/1 -> End Out/1
  Multiport Switch1/1 -> Multiport Switch3/2, Compare To Zero/1, Compare To Zero1/1

== system slib_spectrum_analyser/Preprocessing Window/Direct Memory Access ==
  axim_rd_s2m : Inport
  axim_rd_data : Inport  Port=2
  Length : Inport  Port=3
  Address : Inport  Port=4
  Enable DMA : Inport  Port=5
  Bit Slice : hdlsllib/Logic and Bit Operations/Bit Slice  lidx=0  ridx=0
      settings: SourceProductBaseCode=SL
  Bus Creator : BusCreator  Inputs=3
  Bus Selector1 : BusSelector  OutputSignals=rd_aready,rd_dvalid
  DDR Read Controller : MATLAB Function  TreatAsAtomicUnit=on
  EdgeDetection : Subsystem
  ram_wr_data : Outport  VectorParamsAs1DForOutWhenUnconnected=off
  ram_wr_addr : Outport  Port=2  VectorParamsAs1DForOutWhenUnconnected=off
  ram_wren : Outport  Port=3  VectorParamsAs1DForOutWhenUnconnected=off
  dma_read_ready : Outport  Port=4  VectorParamsAs1DForOutWhenUnconnected=off
  axim_rd_m2s : Outport  Port=5  VectorParamsAs1DForOutWhenUnconnected=off
  wires:
  Enable DMA/1 -> Bit Slice/1
  Address/1 -> DDR Read Controller/2(address)
  DDR Read Controller/4(rd_addr) -> Bus Creator/1  "rd_addr"
  DDR Read Controller/6(rd_avalid) -> Bus Creator/3  "rd_avalid"
  Bus Creator/1 -> axim_rd_m2s/1
  DDR Read Controller/5(rd_len) -> Bus Creator/2  "rd_len"
  Bus Selector1/1 -> DDR Read Controller/4(rd_aready)  "<rd_aready>"
  axim_rd_s2m/1 -> Bus Selector1/1
  Bus Selector1/2 -> DDR Read Controller/5(rd_dvalid)  "<rd_dvalid>"
  axim_rd_data/1 -> ram_wr_data/1
  DDR Read Controller/2(count_out) -> ram_wr_addr/1
  DDR Read Controller/1(valid_out) -> ram_wren/1
  EdgeDetection/1(Out1) -> DDR Read Controller/3(start)
  DDR Read Controller/3(ready_out) -> dma_read_ready/1
  Length/1 -> DDR Read Controller/1(length_in)
  Bit Slice/1 -> EdgeDetection/1(In1)
